simulink model "signum_test"  (Simulink 8.4)
settings: Solver=VariableStepDiscrete  StartTime=0.0  StopTime=0  MaxStep=1  RelTol=1e-3
settings Model: Creator=arnaud  LastModifiedBy=arnaud
settings DataIOCC: ExternalInput=xin  SaveFormat=Structure

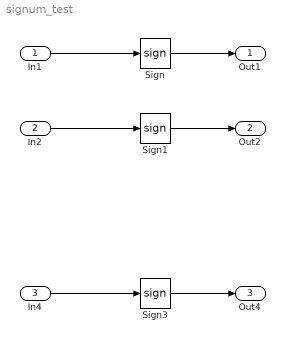
== system signum_test ==
  In1 : Inport  PortDimensions=3
      settings: SignalType=complex
  In2 : Inport  Port=2  PortDimensions=3
  In4 : Inport  Port=3  OutDataTypeStr=int8  PortDimensions=3
  Sign : Signum
  Sign1 : Signum
  Sign3 : Signum
  Out1 : Outport
  Out2 : Outport  Port=2
  Out4 : Outport  Port=3
  wires:
  Sign/1 -> Out1/1
  In1/1 -> Sign/1
  Sign1/1 -> Out2/1
  In2/1 -> Sign1/1
  Sign3/1 -> Out4/1
  In4/1 -> Sign3/1
